simulink library "csc_enf_environmental_forces_lib"  (R2014b)
settings: Solver=ode45  StartTime=0.0  StopTime=10.0  RelTol=1e-3
libraries: util_frame_rotation_lib x1, util_info_lib x1, csu_gsh_gravity_spherical_harmonic_lib x1, csu_prb_orbit_perturbations_model_lib x1
settings Model: Creator=escrane  LastModifiedBy=mstewart

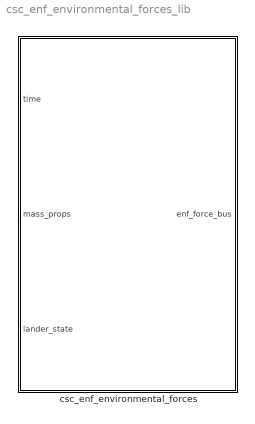
== system csc_enf_environmental_forces_lib ==
  csc_enf_environmental_forces : Subsystem

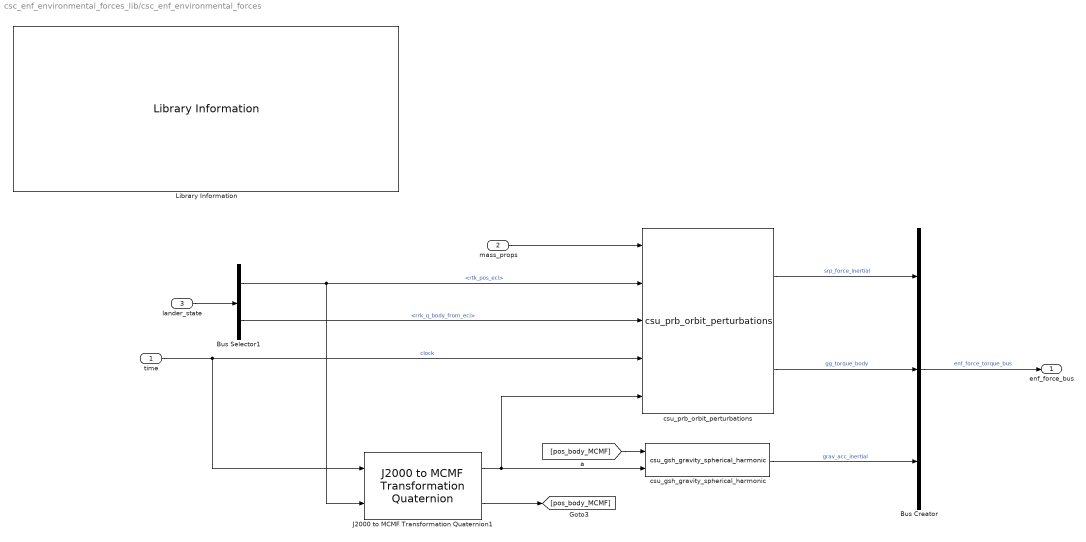
== system csc_enf_environmental_forces_lib/csc_enf_environmental_forces ==
  time : Inport
  mass_props : Inport  Port=2
  lander_state : Inport  Port=3
  Bus Creator : BusCreator  Inputs=3  OutDataTypeStr=Bus: enf_force_torque_msg_t
  Bus Selector1 : BusSelector  OutputSignals=rtk_pos_eci,rrk_q_body_from_eci
  J2000 to MCMF Transformation Quaternion1 : util_frame_rotation_lib/J2000 to MCMF  Transformation Quaternion  SystemSampleTime=-1
  Library Information : util_info_lib/Library Information  owner='escrane'
  csu_gsh_gravity_spherical_harmonic : csu_gsh_gravity_spherical_harmonic_lib/csu_gsh_gravity_spherical_harmonic  mu_central_body=central_body_gravity_mu  r_central_body=central_body_radius
  csu_prb_orbit_perturbations : csu_prb_orbit_perturbations_model_lib/csu_prb_orbit_perturbations
  enf_force_bus : Outport
  wires:
  mass_props/1 -> csu_prb_orbit_perturbations/1
  csu_gsh_gravity_spherical_harmonic/1 -> Bus Creator/3  "grav_acc_inertial"
  csu_prb_orbit_perturbations/2 -> Bus Creator/2  "gg_torque_body"
  csu_prb_orbit_perturbations/1 -> Bus Creator/1  "srp_force_inertial"
  time/1 -> csu_prb_orbit_perturbations/4, J2000 to MCMF Transformation Quaternion1/1  "clock"
  [pos_body_MCMF] -> csu_gsh_gravity_spherical_harmonic/1
  J2000 to MCMF Transformation Quaternion1/2 -> [pos_body_MCMF]
  J2000 to MCMF Transformation Quaternion1/1 -> csu_gsh_gravity_spherical_harmonic/2, csu_prb_orbit_perturbations/5
  Bus Creator/1 -> enf_force_bus/1  "enf_force_torque_bus"
  lander_state/1 -> Bus Selector1/1
  Bus Selector1/1 -> J2000 to MCMF Transformation Quaternion1/2, csu_prb_orbit_perturbations/2  "<rtk_pos_eci>"
  Bus Selector1/2 -> csu_prb_orbit_perturbations/3  "<rrk_q_body_from_eci>"
